simulink model "m080_HeaterAndBucket"  (R2022a)
settings: Solver=VariableStepAuto  StartTime=0.0  StopTime=500  RelTol=1e-3
settings Model: Creator=Admin  LastModifiedBy=Admin

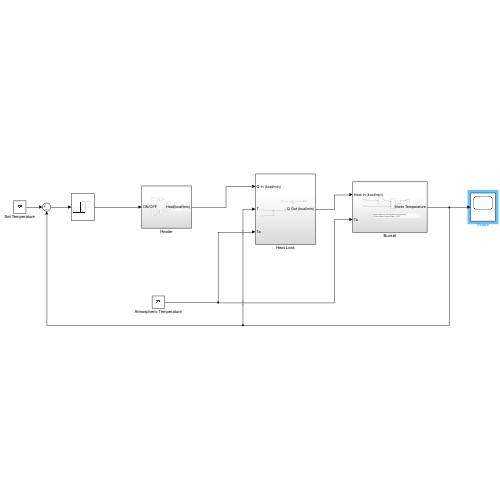
[thumbnail: Simulink's stored preview of the top-level diagram]
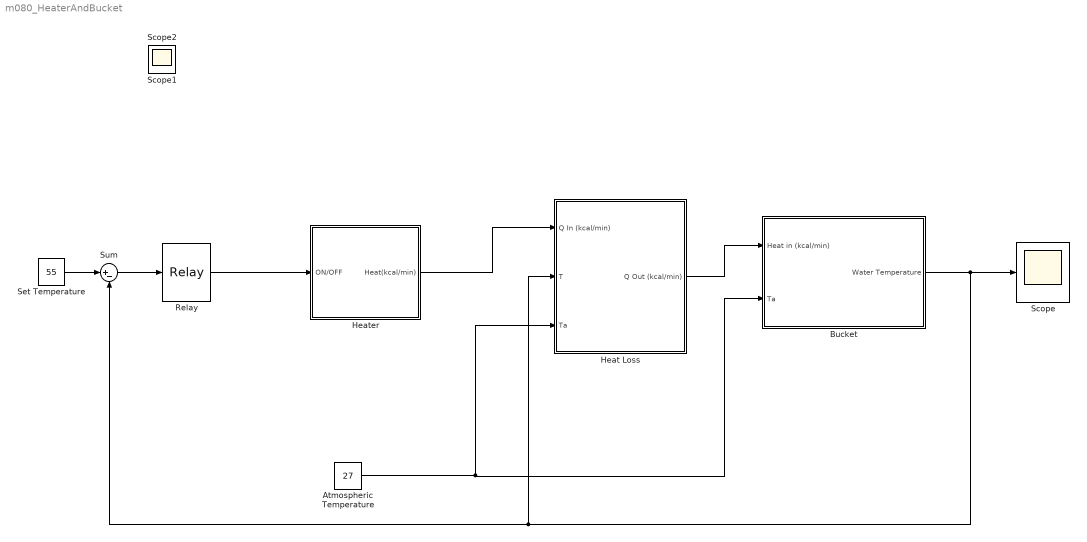
== system m080_HeaterAndBucket ==
  Atmospheric Temperature : Constant  Value=27
  Bucket : Subsystem
  Heat Loss : Subsystem
  Heater : Subsystem
  Relay : Relay  OnSwitchValue=2  OffSwitchValue=-2
  Scope : Scope
  Set Temperature : Constant  Value=55
  Sum : Sum  Inputs=|+-
  Scope1 : Scope
  Scope2 : Scope
  wires:
  Relay/1 -> Heater/1(ON/OFF)
  Heater/1(Heat(kcal/min)) -> Heat Loss/1(Q In (kcal/min))
  Bucket/1(Water Temperature) -> Heat Loss/2(T), Sum/2, Scope/1
  Heat Loss/1(Q Out (kcal/min)) -> Bucket/1(Heat in (kcal/min))
  Atmospheric Temperature/1 -> Bucket/2(Ta), Heat Loss/3(Ta)
  Set Temperature/1 -> Sum/1
  Sum/1 -> Relay/1

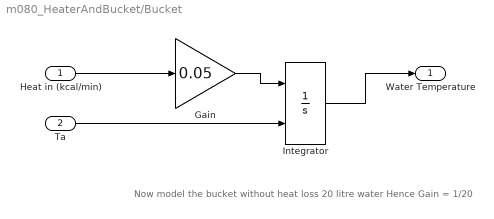
== system m080_HeaterAndBucket/Bucket ==
  note: Now model the bucket without heat loss
      | 20 litre water Hence Gain = 1/20
  Heat in (kcal/min) : Inport
  Ta : Inport  Port=2
  Gain : Gain  Gain=0.05
  Integrator : Integrator  InitialConditionSource=external
  Water Temperature : Outport
  wires:
  Heat in (kcal/min)/1 -> Gain/1
  Gain/1 -> Integrator/1
  Integrator/1 -> Water Temperature/1
  Ta/1 -> Integrator/2

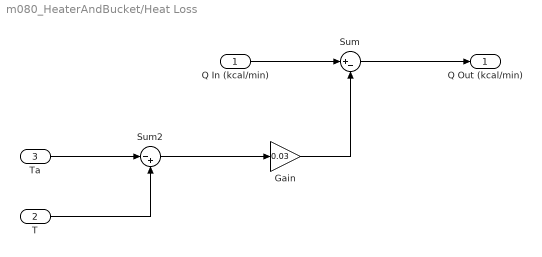
== system m080_HeaterAndBucket/Heat Loss ==
  Q In (kcal/min) : Inport
  T : Inport  Port=2
  Ta : Inport  Port=3
  Gain : Gain  Gain=0.03
  Sum : Sum  Inputs=|+-
  Sum2 : Sum  Inputs=|-+
  Q Out (kcal/min) : Outport
  wires:
  Q In (kcal/min)/1 -> Sum/1
  Sum/1 -> Q Out (kcal/min)/1
  T/1 -> Sum2/2
  Ta/1 -> Sum2/1
  Sum2/1 -> Gain/1
  Gain/1 -> Sum/2

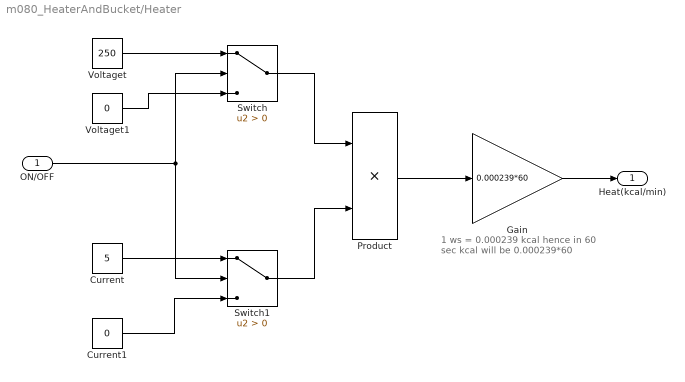
== system m080_HeaterAndBucket/Heater ==
  note: 1 ws = 0.000239 kcal hence
      | in 60 sec kcal will be 0.000239*60
  ON/OFF : Inport
  Current : Constant  Value=5
  Current1 : Constant  Value=0
  Gain : Gain  Gain=0.000239*60
  Product : Product
  Switch : Switch  Criteria=u2 > Threshold  SaturateOnIntegerOverflow=off  InputSameDT=off
  Switch1 : Switch  Criteria=u2 > Threshold  SaturateOnIntegerOverflow=off  InputSameDT=off
  Voltaget : Constant  Value=250
  Voltaget1 : Constant  Value=0
  Heat(kcal/min) : Outport
  wires:
  Gain/1 -> Heat(kcal/min)/1
  Product/1 -> Gain/1
  Voltaget/1 -> Switch/1
  Current/1 -> Switch1/1
  ON/OFF/1 -> Switch1/2, Switch/2
  Voltaget1/1 -> Switch/3
  Switch/1 -> Product/1
  Switch1/1 -> Product/2
  Current1/1 -> Switch1/3
